simulink model "ChiefMaster_TTC580"  (R2022b)
settings: Solver=FixedStepAuto  StartTime=0.0  StopTime=10  FixedStep=0.01  RelTol=1e-3
values from neighbouring files (symbols this model uses):
  BattBox1_No = single(1)    [Parameters.m]
  BattBox2_No = single(2)    [Parameters.m]
  BattBox3_No = single(3)    [Parameters.m]
  CurrentLB = single(-3)    [Parameters.m]
  CurrentReductionConstant_Lvl0 = single(0.03)    [Parameters.m]
  CurrentReductionConstant_Lvl1 = single(0.05)    [Parameters.m]
  CurrentReductionConstant_Lvl2 = single(0.07)    [Parameters.m]
  CurrentReductionConstant_Lvl3 = single(0.1)    [Parameters.m]
  CurrentUB = single(3)    [Parameters.m]
  DCHV_Minus_In_Delay_ms = single(500)    [Parameters.m]
  FL_sHVC_CellBalanceVoltage_mV = single(3500)    [Parameters.m]
  FL_sInrushCurrent_dividebyzero = single(0.00001)    [Parameters.m]
  FL_u8HMI_BuzzerTimer = uint8(3)    [Parameters.m]
  IP_boActValue = true    [Parameters.m]
  IP_boDeactValue = false    [Parameters.m]
  IP_boInitValue = false    [Parameters.m]
  IP_s_LB = 18000    [Parameters.m]
  IP_s_UB = 22000    [Parameters.m]
  IP_sBatt1_ChargeCurrentMax_Factor = single(0.1)    [Parameters.m]
  IP_sBatt1_ChargeCurrentMax_LB = single(0)    [Parameters.m]
  IP_sBatt1_ChargeCurrentMax_Offset = single(0)    [Parameters.m]
  IP_sBatt1_ChargeCurrentMax_UB = single(6553.5)    [Parameters.m]
  IP_sBatt1_Current_Factor = single(0.1)    [Parameters.m]
  IP_sBatt1_Current_LB = single(-3276.8)    [Parameters.m]
  IP_sBatt1_Current_Offset = single(0)    [Parameters.m]
  IP_sBatt1_Current_UB = single(3276.8)    [Parameters.m]
  IP_sBatt1_DisChargeCurrentMax_Factor = single(0.1)    [Parameters.m]
  IP_sBatt1_DisChargeCurrentMax_LB = single(0)    [Parameters.m]
  IP_sBatt1_DisChargeCurrentMax_Offset = single(0)    [Parameters.m]
  IP_sBatt1_DisChargeCurrentMax_UB = single(6553.5)    [Parameters.m]
  IP_sBatt1_InsulationResistance_Factor = single(5)    [Parameters.m]
  IP_sBatt1_InsulationResistance_LB = single(0)    [Parameters.m]
  IP_sBatt1_InsulationResistance_Offset = single(0)    [Parameters.m]
  IP_sBatt1_InsulationResistance_UB = single(0)    [Parameters.m]
  IP_sBatt1_LiBa_IntResist_mOhm = single(25)    [Parameters.m]
  IP_sBatt1_SOC_Factor = single(1)    [Parameters.m]
  IP_sBatt1_SOC_LB = single(0)    [Parameters.m]
  IP_sBatt1_SOC_Offset = single(0)    [Parameters.m]
  IP_sBatt1_SOC_UB = single(100)    [Parameters.m]
  IP_sBatt1_SOH_Factor = single(1)    [Parameters.m]
  IP_sBatt1_SOH_LB = single(0)    [Parameters.m]
  IP_sBatt1_SOH_Offset = single(0)    [Parameters.m]
  IP_sBatt1_SOH_UB = single(100)    [Parameters.m]
  IP_sBatt1_Ubatt_Factor = single(0.1)    [Parameters.m]
  IP_sBatt1_Ubatt_LB = single(0)    [Parameters.m]
  IP_sBatt1_Ubatt_Offset = single(0)    [Parameters.m]
  IP_sBatt1_Ubatt_UB = single(6553.5)    [Parameters.m]
  IP_sBatt1_UserRi_Factor = single(1)    [Parameters.m]
  IP_sBatt1_UserRi_LB = single(0)    [Parameters.m]
  IP_sBatt1_UserRi_Offset = single(0)    [Parameters.m]
  IP_sBatt1_UserRi_UB = single(255)    [Parameters.m]
  IP_sBatt1_VoltageAtSensor_Factor = single(0.02)    [Parameters.m]
  IP_sBatt1_VoltageAtSensor_LB = single(0)    [Parameters.m]
  IP_sBatt1_VoltageAtSensor_Offset = single(0)    [Parameters.m]
  IP_sBatt1_VoltageAtSensor_UB = single(1310.7)    [Parameters.m]
  IP_sBatt2_LiBa_IntResist_mOhm = single(25)    [Parameters.m]
  IP_sBatt3_LiBa_IntResist_mOhm = single(25)    [Parameters.m]
  IP_sEM_LB = 2000    [Parameters.m]
  IP_sEM_UB = 8000    [Parameters.m]
  IP_sFB_LB = 5000    [Parameters.m]
  IP_sFB_UB = 10000    [Parameters.m]
  IP_sHVIL_LB = 12000    [Parameters.m]
  IP_sHVIL_UB = 15000    [Parameters.m]
  IP_sLoad_Voltage_Factor = single(1)    [Parameters.m]
  IP_sLoad_Voltage_LB = single(0)    [Parameters.m]
  IP_sLoad_Voltage_Offset = single(0)    [Parameters.m]
  IP_sLoad_Voltage_UB = single(65535)    [Parameters.m]
  IP_u8HVIL_Delay_ms = uint8(100)    [Parameters.m]
  IP_u8HW_IN_delay_ms = uint8(100)    [Parameters.m]
  IT_sInsulationSafeValue_kOhm = single(650)    [Parameters.m]
  IT_u8IMD_DelayTime_s = uint8(20)    [Parameters.m]
  MainHV_Minus_In_Delay = single(5)    [Parameters.m]
  MainHV_StatusDelay = single(5)    [Parameters.m]
  NotAvailable_uint16 = single(65535)    [Parameters.m]
  NotAvailable_uint8 = uint8(255)    [Parameters.m]
  OP_boHVIL_Supply = boolean(1)    [Parameters.m]
  SafeCurrentToCloseHV_A = single(5)    [Parameters.m]
  SafeVoltageToCloseHV_V = single(0.5)    [Parameters.m]
  UnexpectedBattChargingFcn_Available = boolean(1)    [Parameters.m]
  Voltage_NA_UB = uint16(65535)    [Parameters.m]
  VoltageSensorAvailableBB1 = boolean(0)    [Parameters.m]
  VoltageSensorAvailableBB2 = boolean(0)    [Parameters.m]
  VoltageSensorAvailableBB3 = boolean(0)    [Parameters.m]
libraries: simulink x184, Library_DataProcessing_v1_1 x167, Library_DataProcessing_v1 x142, libCM x28
(part 6 of 19)

== system ChiefMaster_TTC580/ChiefMaster/Flow Logic/System Status/Subsystem1 ==
  IP_boBMS_SDError_BB1 : Inport
  IP_boBMS_SDError_BB2 : Inport  Port=2
  IP_boBMS_SDError_BB3 : Inport  Port=3
  IP_boBMS_HV_REL_ON_BB1 : Inport  Port=4
  IP_boBMS_HV_REL_ON_BB2 : Inport  Port=5
  IP_boBMS_HV_REL_ON_BB3 : Inport  Port=6
  Add : Sum  Inputs=++++++
  Constant : Constant  Value=0  OutDataTypeStr=boolean
  Constant1 : Constant  Value=0  OutDataTypeStr=boolean
  OR : Logic  Operator=OR  Inputs=3  AllPortsSameDT=off  OutDataTypeStr=boolean
  Switch : Switch  Criteria=u2 > Threshold  SaturateOnIntegerOverflow=off  InputSameDT=off
  Switch1 : Switch  Criteria=u2 > Threshold  SaturateOnIntegerOverflow=off  InputSameDT=off
  Switch2 : Switch  Criteria=u2 > Threshold  SaturateOnIntegerOverflow=off  InputSameDT=off
  FL_boSS_System_Error : Outport
  FL_u8SS_System_ErrorCode : Outport  Port=2
  wires:
  IP_boBMS_SDError_BB1/1 -> Switch/1
  IP_boBMS_SDError_BB2/1 -> Switch1/1
  IP_boBMS_SDError_BB3/1 -> Switch2/1
  OR/1 -> FL_boSS_System_Error/1  "FL_boSS_System_Error"
  IP_boBMS_HV_REL_ON_BB1/1 -> Switch/2
  Constant/1 -> Switch/3, Switch2/3, Switch1/3
  IP_boBMS_HV_REL_ON_BB2/1 -> Switch1/2
  IP_boBMS_HV_REL_ON_BB3/1 -> Switch2/2
  Add/1 -> FL_u8SS_System_ErrorCode/1  "FL_u8SS_System_ErrorCode"
  Switch2/1 -> Add/3, OR/3
  Switch/1 -> Add/1, OR/1
  Constant1/1 -> Add/4, Add/5, Add/6
  Switch1/1 -> Add/2, OR/2

== system ChiefMaster_TTC580/ChiefMaster/Flow Logic/System Status/Subsystem2 ==
  BatteryPackSignals : Inport
  Bus Selector : BusSelector  OutputSignals=IT_BatterySignal_Databus.IT_u8BMS_SOC_BB1,IT_BatterySignal_Databus.IT_boBMS_HV_REL_ON_BB1,IT_BatterySignal_Databus.IT_u8BMS_SOC_BB2,IT_BatterySignal_Databus.IT_boBMS_HV_REL_ON_BB2,IT_BatterySignal_Databus.IT_u8BMS_SOC_BB3,IT_BatterySignal_Databus.IT_boBMS_HV_REL_ON_BB3
  Constant : Constant  Value=NotAvailable_uint8  OutDataTypeStr=uint8
  Constant1 : Constant  Value=0  OutDataTypeStr=uint8
  Data Type Conversion : DataTypeConversion  OutDataTypeStr=uint8  SaturateOnIntegerOverflow=off  RndMeth=Floor
  Data Type Conversion1 : DataTypeConversion  OutDataTypeStr=uint8  SaturateOnIntegerOverflow=off  RndMeth=Floor
  Data Type Conversion2 : DataTypeConversion  OutDataTypeStr=uint8  SaturateOnIntegerOverflow=off  RndMeth=Floor
  Min : MinMax  Inputs=3
  OR : Logic  Operator=OR  Inputs=3  AllPortsSameDT=off  OutDataTypeStr=boolean
  Switch{,1..3} (4 alike) : Switch  Criteria=u2 > Threshold  SaturateOnIntegerOverflow=off  InputSameDT=off
  FL_u8SS_SystemSOC : Outport
  wires:
  Min/1 -> FL_u8SS_SystemSOC/1
  Bus Selector/6 -> OR/1, Switch2/2  "<IT_boBMS_HV_REL_ON_BB3>"
  Bus Selector/2 -> OR/3, Switch/2  "<IT_boBMS_HV_REL_ON_BB1>"
  Bus Selector/4 -> OR/2, Switch1/2  "<IT_boBMS_HV_REL_ON_BB2>"
  Switch2/1 -> Min/3
  Switch/1 -> Min/1
  Bus Selector/1 -> Data Type Conversion/1  "<IT_u8BMS_SOC_BB1>"
  Switch1/1 -> Min/2
  Bus Selector/3 -> Data Type Conversion1/1  "<IT_u8BMS_SOC_BB2>"
  Bus Selector/5 -> Data Type Conversion2/1  "<IT_u8BMS_SOC_BB3>"
  Switch3/1 -> Switch2/3, Switch/3, Switch1/3
  OR/1 -> Switch3/2
  Constant/1 -> Switch3/1
  Constant1/1 -> Switch3/3
  BatteryPackSignals/1 -> Bus Selector/1
  Data Type Conversion/1 -> Switch/1
  Data Type Conversion1/1 -> Switch1/1
  Data Type Conversion2/1 -> Switch2/1

== system ChiefMaster_TTC580/ChiefMaster/Flow Logic/System Status/Subsystem3 ==
  BatteryPackSignals : Inport
  Add : Sum  Inputs=+++
  Bus Selector : BusSelector  OutputSignals=IT_BatterySignal_Databus.IT_sBMS_Current_BB1,IT_BatterySignal_Databus.IT_sBMS_Current_BB2,IT_BatterySignal_Databus.IT_sBMS_Current_BB3
  FL_sSS_System_Current : Outport
  wires:
  Bus Selector/3 -> Add/3  "<IT_sBMS_Current_BB3>"
  Bus Selector/2 -> Add/2  "<IT_sBMS_Current_BB2>"
  Bus Selector/1 -> Add/1  "<IT_sBMS_Current_BB1>"
  Add/1 -> FL_sSS_System_Current/1
  BatteryPackSignals/1 -> Bus Selector/1

== system ChiefMaster_TTC580/ChiefMaster/Flow Logic/System Status/Subsystem4 ==
  BatteryPackSignals : Inport
  Bus Selector : BusSelector  OutputSignals=IT_BatterySignal_Databus.IT_sBMS_VtgInt_BB1,IT_BatterySignal_Databus.IT_boBMS_HV_REL_ON_BB1,IT_BatterySignal_Databus.IT_sBMS_VtgInt_BB2,IT_BatterySignal_Databus.IT_boBMS_HV_REL_ON_BB2,IT_BatterySignal_Databus.IT_sBMS_VtgInt_BB3,IT_BatterySignal_Databus.IT_boBMS_HV_REL_ON_BB3
  Constant : Constant  Value=0  OutDataTypeStr=single
  Min : MinMax  Function=max  Inputs=3
  Switch : Switch  Criteria=u2 > Threshold  SaturateOnIntegerOverflow=off  InputSameDT=off
  Switch1 : Switch  Criteria=u2 > Threshold  SaturateOnIntegerOverflow=off  InputSameDT=off
  Switch2 : Switch  Criteria=u2 > Threshold  SaturateOnIntegerOverflow=off  InputSameDT=off
  FL_sST_SystemVoltage : Outport
  wires:
  BatteryPackSignals/1 -> Bus Selector/1
  Min/1 -> FL_sST_SystemVoltage/1
  Bus Selector/6 -> Switch2/2  "<IT_boBMS_HV_REL_ON_BB3>"
  Bus Selector/2 -> Switch/2  "<IT_boBMS_HV_REL_ON_BB1>"
  Bus Selector/4 -> Switch1/2  "<IT_boBMS_HV_REL_ON_BB2>"
  Switch2/1 -> Min/3
  Switch/1 -> Min/1
  Bus Selector/1 -> Switch/1  "<IT_sBMS_VtgInt_BB1>"
  Switch1/1 -> Min/2
  Bus Selector/3 -> Switch1/1  "<IT_sBMS_VtgInt_BB2>"
  Bus Selector/5 -> Switch2/1  "<IT_sBMS_VtgInt_BB3>"
  Constant/1 -> Switch/3, Switch1/3, Switch2/3

== system ChiefMaster_TTC580/ChiefMaster/Flow Logic/System Status/Subsystem7 ==
  IP_boBMS_HV_REL_ON_BB1 : Inport
  IP_boBMS_HV_REL_ON_BB2 : Inport  Port=2
  IP_boBMS_HV_REL_ON_BB3 : Inport  Port=3
  FL_u8Sig_No_Of_Batt_Usable : Inport  Port=4
  IP_boBMS_SDError_BB1 : Inport  Port=5
  IP_boBMS_SDError_BB2 : Inport  Port=6
  IP_boBMS_SDError_BB3 : Inport  Port=7
  AND : Logic  Inputs=4  AllPortsSameDT=off  OutDataTypeStr=boolean
  AND1 : Logic  Inputs=4  AllPortsSameDT=off  OutDataTypeStr=boolean
  AND2 : Logic  Inputs=4  AllPortsSameDT=off  OutDataTypeStr=boolean
  Add : Sum  Inputs=+++
  Compare To Constant : simulink/Logic and Bit Operations/Compare To Constant  relop===  const=1  OutDataTypeStr=boolean
  Compare To Constant1 : simulink/Logic and Bit Operations/Compare To Constant  relop=>  const=0  OutDataTypeStr=boolean
  OR3 : Logic  Operator=OR  Inputs=3  AllPortsSameDT=off  OutDataTypeStr=boolean
  Unit Delay : UnitDelay  SampleTime=-1  HasFrameUpgradeWarning=on
  Unit Delay1 : UnitDelay  SampleTime=-1  HasFrameUpgradeWarning=on
  Unit Delay2 : UnitDelay  SampleTime=-1  HasFrameUpgradeWarning=on
  FL_u8SS_NumberOfConnectedBatt : Outport
  FL_boSS_BDU_Reset : Outport  Port=2
  wires:
  Compare To Constant1/1 -> AND2/3, AND1/1, AND/3
  AND/1 -> OR3/1  "BDU_Reset"
  Compare To Constant/1 -> AND1/2, AND2/2, AND/2
  AND2/1 -> OR3/3  "BDU_Reset"
  Unit Delay1/1 -> AND1/4
  IP_boBMS_HV_REL_ON_BB2/1 -> Add/2, AND1/3
  FL_u8Sig_No_Of_Batt_Usable/1 -> Compare To Constant1/1
  IP_boBMS_HV_REL_ON_BB1/1 -> Add/1, AND/1
  Add/1 -> FL_u8SS_NumberOfConnectedBatt/1, Compare To Constant/1  "FL_u8SS_NumberOfConnectedBatt"
  IP_boBMS_HV_REL_ON_BB3/1 -> AND2/1, Add/3
  AND1/1 -> OR3/2  "BDU_Reset"
  Unit Delay/1 -> AND/4
  Unit Delay2/1 -> AND2/4
  OR3/1 -> FL_boSS_BDU_Reset/1  "FL_boSS_BDU_Reset"
  IP_boBMS_SDError_BB3/1 -> Unit Delay2/1
  IP_boBMS_SDError_BB1/1 -> Unit Delay/1
  IP_boBMS_SDError_BB2/1 -> Unit Delay1/1

== system ChiefMaster_TTC580/ChiefMaster/Flow Logic/System Status/Subsystem8 ==
  <FL_boREQ_IMD_ON_BB1> : Inport
  <FL_boREQ_IMD_ON_BB2> : Inport  Port=2
  <FL_boREQ_IMD_ON_BB3> : Inport  Port=3
  AND : Logic  Inputs=3  AllPortsSameDT=off  OutDataTypeStr=boolean
  Unit Delay7 : UnitDelay  SampleTime=-1  HasFrameUpgradeWarning=on
  Unit Delay8 : UnitDelay  SampleTime=-1  HasFrameUpgradeWarning=on
  Unit Delay9 : UnitDelay  SampleTime=-1  HasFrameUpgradeWarning=on
  REQ_IMD_ON : Outport
  wires:
  <FL_boREQ_IMD_ON_BB3>/1 -> Unit Delay7/1
  <FL_boREQ_IMD_ON_BB1>/1 -> Unit Delay9/1
  <FL_boREQ_IMD_ON_BB2>/1 -> Unit Delay8/1
  AND/1 -> REQ_IMD_ON/1
  Unit Delay9/1 -> AND/1
  Unit Delay8/1 -> AND/2
  Unit Delay7/1 -> AND/3

== system ChiefMaster_TTC580/ChiefMaster/Input Processing/Actia/Batt Box 1 ==
  C_Actia_Batt1_MyStatus : Inport
  C_Actia_Batt1_MyStatus_Timeout : Inport  Port=2  OutDataTypeStr=boolean
  C_Actia_Batt1_Error : Inport  Port=3
  C_Actia_Batt1_Error_Timeout : Inport  Port=4  OutDataTypeStr=boolean
  C_Actia_Batt1_ADS_8 : Inport  Port=5
  C_Actia_Batt1_ADS_8_Timeout : Inport  Port=6  OutDataTypeStr=boolean
  C_Actia_Batt1_ADS_0 : Inport  Port=7
  C_Actia_Batt1_ADS_0_Timeout : Inport  Port=8
  C_Actia_Batt1_ADS_1 : Inport  Port=9
  C_Actia_Batt1_ADS_1_Timeout : Inport  Port=10  OutDataTypeStr=boolean
  C_Actia_Batt1_ADS_3 : Inport  Port=11
  C_Actia_Batt1_ADS_3_Timeout : Inport  Port=12
  Bus Creator : BusCreator  Inputs=17
  Subsystem1 : Subsystem
  Subsystem13 : Subsystem
  Subsystem2 : Subsystem
  Subsystem3 : Subsystem
  Subsystem4 : Subsystem
  Subsystem5 : Subsystem
  Subsystem6 : Subsystem
  IP_Actia_Batt1_Databus : Outport
  wires:
  Subsystem2/3(IP_sActia_Batt1_DisChargeCurrentMax_A_Databus) -> Bus Creator/3
  Subsystem5/3(IP_sActia_Batt1_SOC_percent_DataBus) -> Bus Creator/9
  Subsystem4/1(IP_Actia_sBatt1_MyStatus2_Databus) -> Bus Creator/5
  C_Actia_Batt1_ADS_1_Timeout/1 -> Subsystem13/5(C_Batt1_ADS_1_520_Timeout), Subsystem6/2(C_Batt1_ADS_1_520_Timeout)
  C_Actia_Batt1_MyStatus_Timeout/1 -> Subsystem13/1(C_Batt1_MyStatus_140_Timeout), Subsystem2/2(C_Actia_Batt1_MyStatus_Timeout)
  C_Actia_Batt1_ADS_1/1 -> Subsystem6/1(C_Batt1_ADS_1_520)
  C_Actia_Batt1_ADS_3_Timeout/1 -> Subsystem13/6(C_Batt1_ADS_3_560_Timeout), Subsystem1/2(C_Batt1_ADS_3_560_Timeout)
  C_Actia_Batt1_Error_Timeout/1 -> Subsystem4/2(C_Actia_Batt1_Error_Timeout), Subsystem13/2(C_Batt1_Error_100_Timeout)
  C_Actia_Batt1_ADS_8/1 -> Subsystem5/1(C_Batt1_ADS_8_600)
  Subsystem6/1(IP_sActia_Batt1_UserRi_mOhms_DataBus) -> Bus Creator/13
  Subsystem1/1(IP_sActia_Batt1_Ubatt_Databus) -> Bus Creator/16
  Subsystem5/2(IP_sActia_Batt1_InsulationResistance_kOhms_DataBus) -> Bus Creator/8
  Subsystem2/4(IP_sActia_Batt1_VoltageAtSensor_V_Databus) -> Bus Creator/4
  Subsystem2/2(IP_sActia_Batt1_ChargeCurrentMax_A_Databus) -> Bus Creator/2
  C_Actia_Batt1_ADS_8_Timeout/1 -> Subsystem13/3(C_Batt1_ADS_8_600_Timeout), Subsystem5/2(C_Batt1_ADS_8_600_Timeout)
  Subsystem5/1(IP_sActia_Batt1_Current_A_DataBus) -> Bus Creator/7
  Subsystem5/4(IP_sActia_Batt1_SOH_percent_DataBus) -> Bus Creator/10
  Subsystem2/1(Batt1_MyStatus1_Databus) -> Bus Creator/1
  Subsystem13/1(IP_sActia_Batt1_Availability) -> Bus Creator/17
  Bus Creator/1 -> IP_Actia_Batt1_Databus/1  "IP_Actia_Batt1_Databus"
  C_Actia_Batt1_ADS_3/1 -> Subsystem1/1(C_Batt1_ADS_3_560)
  C_Actia_Batt1_MyStatus/1 -> Subsystem2/1(C_Actia_Batt1_MyStatus_Msg)
  C_Actia_Batt1_Error/1 -> Subsystem4/1(C_Actia_Batt1_Error)
  Subsystem4/2(IP_Actia_Batt1_Error_Databus) -> Bus Creator/6
  Subsystem6/2(IP_sActia_Batt1_MinTemp_degC_DataBus) -> Bus Creator/14
  Subsystem6/3(IP_sActia_Batt1_MaxTemp_degC_DataBus) -> Bus Creator/15
  C_Actia_Batt1_ADS_0/1 -> Subsystem3/1(C_Batt1_ADS_0_500)
  C_Actia_Batt1_ADS_0_Timeout/1 -> Subsystem13/4(C_Batt1_ADS_0_500_Timeout), Subsystem3/2(C_Batt1_ADS_0_500_Timeout)
  Subsystem3/1(IP_sActia_Batt1_MinCellVolt_mV_DataBus) -> Bus Creator/11
  Subsystem3/2(IP_sActia_Batt1_MaxCellVolt_mV_DataBus) -> Bus Creator/12

== system ChiefMaster_TTC580/ChiefMaster/Input Processing/Actia/Batt Box 2 ==
  C_Actia_Batt2_MyStatus : Inport
  C_Actia_Batt2_MyStatus_Timeout : Inport  Port=2  OutDataTypeStr=boolean
  C_Actia_Batt2_Error : Inport  Port=3
  C_Actia_Batt2_Error_Timeout : Inport  Port=4  OutDataTypeStr=boolean
  C_Actia_Batt2_ADS_8 : Inport  Port=5
  C_Actia_Batt2_ADS_8_Timeout : Inport  Port=6  OutDataTypeStr=boolean
  C_Actia_Batt2_ADS_0 : Inport  Port=7
  C_Actia_Batt2_ADS_0_Timeout : Inport  Port=8
  C_Actia_Batt2_ADS_1 : Inport  Port=9
  C_Actia_Batt2_ADS_1_Timeout : Inport  Port=10  OutDataTypeStr=boolean
  C_Actia_Batt2_ADS_3 : Inport  Port=11
  C_Actia_Batt2_ADS_3_Timeout : Inport  Port=12
  Bus Creator : BusCreator  Inputs=17
  Subsystem1 : Subsystem
  Subsystem13 : Subsystem
  Subsystem2 : Subsystem
  Subsystem3 : Subsystem
  Subsystem4 : Subsystem
  Subsystem5 : Subsystem
  Subsystem6 : Subsystem
  IP_Actia_Batt2_Databus : Outport
  wires:
  Subsystem4/2(IP_Actia_Batt2_Error_Databus) -> Bus Creator/6
  C_Actia_Batt2_Error/1 -> Subsystem4/1(C_Actia_Batt2_Error)
  C_Actia_Batt2_MyStatus/1 -> Subsystem2/1(C_Actia_Batt2_MyStatus_Msg)
  C_Actia_Batt2_ADS_3/1 -> Subsystem1/1(C_Batt2_ADS_3_560)
  Bus Creator/1 -> IP_Actia_Batt2_Databus/1  "IP_Actia_Batt2_Databus"
  Subsystem13/1(IP_sActia_Batt2_Availability) -> Bus Creator/17
  Subsystem2/1(Batt2_MyStatus1_Databus) -> Bus Creator/1
  Subsystem5/4(IP_sActia_Batt2_SOH_percent_DataBus) -> Bus Creator/10
  Subsystem5/1(IP_sActia_Batt2_Current_A_DataBus) -> Bus Creator/7
  C_Actia_Batt2_ADS_8_Timeout/1 -> Subsystem5/2(C_Batt2_ADS_8_600_Timeout), Subsystem13/3(C_Batt2_ADS_8_600_Timeout)
  Subsystem2/2(IP_sActia_Batt2_ChargeCurrentMax_A_Databus) -> Bus Creator/2
  Subsystem2/4(IP_sActia_Batt2_VoltageAtSensor_V_Databus) -> Bus Creator/4
  Subsystem5/2(IP_sActia_Batt2_InsulationResistance_kOhms_DataBus) -> Bus Creator/8
  Subsystem1/1(IP_sActia_Batt2_Ubatt_Databus) -> Bus Creator/16
  Subsystem6/1(IP_sActia_Batt2_UserRi_mOhms_DataBus) -> Bus Creator/13
  C_Actia_Batt2_ADS_8/1 -> Subsystem5/1(C_Batt2_ADS_8_600)
  C_Actia_Batt2_Error_Timeout/1 -> Subsystem4/2(C_Actia_Batt2_Error_Timeout), Subsystem13/2(C_Batt2_Error_100_Timeout)
  C_Actia_Batt2_ADS_3_Timeout/1 -> Subsystem1/2(C_Batt2_ADS_3_560_Timeout), Subsystem13/6(C_Batt2_ADS_3_560_Timeout)
  C_Actia_Batt2_ADS_1/1 -> Subsystem6/1(C_Batt2_ADS_1_520)
  C_Actia_Batt2_MyStatus_Timeout/1 -> Subsystem2/2(C_Actia_Batt2_MyStatus_Timeout), Subsystem13/1(C_Batt2_MyStatus_140_Timeout)
  C_Actia_Batt2_ADS_1_Timeout/1 -> Subsystem6/2(C_Batt2_ADS_1_520_Timeout), Subsystem13/5(C_Batt2_ADS_1_520_Timeout)
  Subsystem4/1(IP_Actia_sBatt2_MyStatus2_Databus) -> Bus Creator/5
  Subsystem5/3(IP_sActia_Batt2_SOC_percent_DataBus) -> Bus Creator/9
  Subsystem2/3(IP_sActia_Batt2_DisChargeCurrentMax_A_Databus) -> Bus Creator/3
  Subsystem6/2(IP_sActia_Batt2_MinTemp_degC_DataBus) -> Bus Creator/14
  Subsystem6/3(IP_sActia_Batt2_MaxTemp_degC_DataBus) -> Bus Creator/15
  C_Actia_Batt2_ADS_0_Timeout/1 -> Subsystem13/4(C_Batt2_ADS_501_Timeout), Subsystem3/2(C_Batt1_ADS_0_500_Timeout)
  Subsystem3/2(IP_sActia_Batt2_MaxCellVolt_mV_DataBus) -> Bus Creator/12
  Subsystem3/1(IP_sActia_Batt2_MinCellVolt_mV_DataBus) -> Bus Creator/11
  C_Actia_Batt2_ADS_0/1 -> Subsystem3/1(C_Batt1_ADS_0_500)

== system ChiefMaster_TTC580/ChiefMaster/Input Processing/Actia/Batt Box 3 ==
  C_Actia_Batt3_MyStatus : Inport
  C_Actia_Batt3_MyStatus_Timeout : Inport  Port=2
  C_Actia_Batt3_Error : Inport  Port=3
  C_Actia_Batt3_Error_Timeout : Inport  Port=4
  C_Actia_Batt3_ADS_8 : Inport  Port=5
  C_Actia_Batt3_ADS_8_Timeout : Inport  Port=6
  C_Actia_Batt3_ADS_0 : Inport  Port=7
  C_Actia_Batt3_ADS_0_Timeout : Inport  Port=8
  C_Actia_Batt3_ADS_1 : Inport  Port=9
  C_Actia_Batt3_ADS_1_Timeout : Inport  Port=10
  C_Actia_Batt3_ADS_3 : Inport  Port=11
  C_Actia_Batt3_ADS_3_Timeout : Inport  Port=12
  Bus Creator : BusCreator  Inputs=17
  Subsystem1 : Subsystem
  Subsystem13 : Subsystem
  Subsystem2 : Subsystem
  Subsystem3 : Subsystem
  Subsystem4 : Subsystem
  Subsystem5 : Subsystem
  Subsystem6 : Subsystem
  IP_Actia_Batt3_Databus : Outport
  wires:
  Subsystem2/3(IP_sActia_Batt3_DisChargeCurrentMax_A_Databus) -> Bus Creator/3
  Subsystem5/3(IP_sActia_Batt3_SOC_percent_DataBus) -> Bus Creator/9
  Subsystem4/1(IP_Actia_sBatt3_MyStatus2_Databus) -> Bus Creator/5
  C_Actia_Batt3_ADS_1_Timeout/1 -> Subsystem13/5(C_Batt3_ADS_1_520_Timeout), Subsystem6/2(C_Batt3_ADS_1_520_Timeout)
  C_Actia_Batt3_MyStatus_Timeout/1 -> Subsystem13/1(C_Batt3_MyStatus_140_Timeout), Subsystem2/2(C_Actia_Batt3_MyStatus_Timeout)
  C_Actia_Batt3_ADS_1/1 -> Subsystem6/1(C_Batt3_ADS_1_520)
  C_Actia_Batt3_ADS_3_Timeout/1 -> Subsystem13/6(C_Batt3_ADS_3_560_Timeout), Subsystem1/2(C_Batt3_ADS_3_560_Timeout)
  C_Actia_Batt3_Error_Timeout/1 -> Subsystem4/2(C_Actia_Batt3_Error_Timeout), Subsystem13/2(C_Batt3_Error_100_Timeout)
  C_Actia_Batt3_ADS_8/1 -> Subsystem5/1(C_Batt3_ADS_8_600)
  Subsystem6/1(IP_sActia_Batt3_UserRi_mOhms_DataBus) -> Bus Creator/13
  Subsystem1/1(IP_sActia_Batt3_Ubatt_Databus) -> Bus Creator/16
  Subsystem5/2(IP_sActia_Batt3_InsulationResistance_kOhms_DataBus) -> Bus Creator/8
  Subsystem2/4(IP_sActia_Batt3_VoltageAtSensor_V_Databus) -> Bus Creator/4
  Subsystem2/2(IP_sActia_Batt3_ChargeCurrentMax_A_Databus) -> Bus Creator/2
  C_Actia_Batt3_ADS_8_Timeout/1 -> Subsystem5/2(C_Batt3_ADS_8_600_Timeout), Subsystem13/3(C_Batt3_ADS_8_600_Timeout)
  Subsystem5/1(IP_sActia_Batt3_Current_A_DataBus) -> Bus Creator/7
  Subsystem5/4(IP_sActia_Batt3_SOH_percent_DataBus) -> Bus Creator/10
  Subsystem2/1(Batt3_MyStatus1_Databus) -> Bus Creator/1
  Subsystem13/1(IP_sActia_Batt3_Availability) -> Bus Creator/17
  Bus Creator/1 -> IP_Actia_Batt3_Databus/1  "IP_Actia_Batt3_Databus"
  C_Actia_Batt3_ADS_3/1 -> Subsystem1/1(C_Batt3_ADS_3_560)
  C_Actia_Batt3_MyStatus/1 -> Subsystem2/1(C_Actia_Batt3_MyStatus_Msg)
  C_Actia_Batt3_Error/1 -> Subsystem4/1(C_Actia_Batt3_Error)
  Subsystem4/2(IP_Actia_Batt3_Error_Databus) -> Bus Creator/6
  Subsystem6/2(IP_sActia_Batt3_MinTemp_degC_DataBus) -> Bus Creator/14
  Subsystem6/3(IP_sActia_Batt3_MaxTemp_degC_DataBus) -> Bus Creator/15
  C_Actia_Batt3_ADS_0_Timeout/1 -> Subsystem13/4(C_Batt2_ADS_0_Timeout), Subsystem3/2(C_Batt1_ADS_0_500_Timeout)
  C_Actia_Batt3_ADS_0/1 -> Subsystem3/1(C_Batt1_ADS_0_500)
  Subsystem3/1(IP_sActia_Batt3_MinCellVolt_mV_DataBus) -> Bus Creator/11
  Subsystem3/2(IP_sActia_Batt3_MaxCellVolt_mV_DataBus) -> Bus Creator/12

== system ChiefMaster_TTC580/ChiefMaster/Input Processing/HW Inputs/EmergencyButtonNC ==
  "EmergencyButton_NC " : Inport  OutDataTypeStr=single
  Constant : Constant  Value=IP_sEM_LB  OutDataTypeStr=single
  Constant1 : Constant  Value=IP_sEM_UB  OutDataTypeStr=single
  Constant2 : Constant  Value=IP_boActValue  OutDataTypeStr=boolean
  Constant3 : Constant  Value=IP_boDeactValue  OutDataTypeStr=boolean
  Constant4 : Constant  Value=IP_boInitValue  OutDataTypeStr=boolean
  Lib_Hysteresis_HighActive : Library_DataProcessing_v1_1/Lib_Hysteresis_HighActive  SystemSampleTime=-1  VariantActivationTime=update diagram  Latency=0  AutoFrameSizeCalculation=off
  IP_boHW_EmergencyButton_NC : Outport
  wires:
  Lib_Hysteresis_HighActive/1 -> IP_boHW_EmergencyButton_NC/1  "IP_boHW_EmergencyButton_NC"
  Constant1/1 -> Lib_Hysteresis_HighActive/6
  Constant/1 -> Lib_Hysteresis_HighActive/5
  Constant3/1 -> Lib_Hysteresis_HighActive/4
  Constant2/1 -> Lib_Hysteresis_HighActive/3
  Constant4/1 -> Lib_Hysteresis_HighActive/2
  "EmergencyButton_NC "/1 -> Lib_Hysteresis_HighActive/1

== system ChiefMaster_TTC580/ChiefMaster/Input Processing/HW Inputs/EmergencyButtonNO ==
  "EmergencyButton_NO " : Inport  OutDataTypeStr=single
  Constant : Constant  Value=IP_s_UB  OutDataTypeStr=single
  Constant1 : Constant  Value=IP_s_LB  OutDataTypeStr=single
  Constant2 : Constant  Value=IP_boActValue  OutDataTypeStr=boolean
  Constant3 : Constant  Value=IP_boDeactValue  OutDataTypeStr=boolean
  Constant4 : Constant  Value=IP_boInitValue  OutDataTypeStr=boolean
  Lib_Hysteresis_HighActive : Library_DataProcessing_v1_1/Lib_Hysteresis_HighActive  SystemSampleTime=-1  VariantActivationTime=update diagram  Latency=0  AutoFrameSizeCalculation=off
  IP_boHW_EmergencyButton_NO : Outport
  wires:
  "EmergencyButton_NO "/1 -> Lib_Hysteresis_HighActive/1
  Constant4/1 -> Lib_Hysteresis_HighActive/2
  Constant2/1 -> Lib_Hysteresis_HighActive/3
  Constant3/1 -> Lib_Hysteresis_HighActive/4
  Constant/1 -> Lib_Hysteresis_HighActive/6
  Constant1/1 -> Lib_Hysteresis_HighActive/5
  Lib_Hysteresis_HighActive/1 -> IP_boHW_EmergencyButton_NO/1  "IP_boHW_EmergencyButton_NO"

== system ChiefMaster_TTC580/ChiefMaster/Input Processing/HW Inputs/HVIL ==
  IP_sHW_HVIL_BDU : Inport
  Constant : Constant  Value=IP_sHVIL_UB  OutDataTypeStr=single
  Constant1 : Constant  Value=IP_sHVIL_LB  OutDataTypeStr=single
  Constant2 : Constant  Value=IP_boActValue  OutDataTypeStr=boolean
  Constant3 : Constant  Value=IP_boDeactValue  OutDataTypeStr=boolean
  Constant4 : Constant  Value=IP_boInitValue  OutDataTypeStr=boolean
  Constant5 : Constant  Value=IP_u8HVIL_Delay_ms  OutDataTypeStr=uint8
  HVIL_Input_Delay : Stateflow chart  TreatAsAtomicUnit=on
  Lib_Hysteresis_HighActive : Library_DataProcessing_v1_1/Lib_Hysteresis_HighActive  SystemSampleTime=-1  VariantActivationTime=update diagram  Latency=0  AutoFrameSizeCalculation=off
  IP_boHW_HVIL_BDU : Outport
  wires:
  Constant4/1 -> Lib_Hysteresis_HighActive/2
  Constant2/1 -> Lib_Hysteresis_HighActive/3
  Constant3/1 -> Lib_Hysteresis_HighActive/4
  Constant1/1 -> Lib_Hysteresis_HighActive/5
  Constant/1 -> Lib_Hysteresis_HighActive/6
  IP_sHW_HVIL_BDU/1 -> Lib_Hysteresis_HighActive/1
  HVIL_Input_Delay/1(out) -> IP_boHW_HVIL_BDU/1  "IP_boHW_HVIL_BDU"
  Lib_Hysteresis_HighActive/1 -> HVIL_Input_Delay/1(HVIL_IN)  "IP_boHW_HVIL_BDU"
  Constant5/1 -> HVIL_Input_Delay/2(IP_HVIL_Delay_ms)

== system ChiefMaster_TTC580/ChiefMaster/Input Processing/HW Inputs/HVIL1 ==
  IP_sHW_HVIL_BDU : Inport
  Constant : Constant  Value=IP_sHVIL_UB  OutDataTypeStr=single
  Constant1 : Constant  Value=IP_sHVIL_LB  OutDataTypeStr=single
  Constant2 : Constant  Value=IP_boActValue  OutDataTypeStr=boolean
  Constant3 : Constant  Value=IP_boDeactValue  OutDataTypeStr=boolean
  Constant4 : Constant  Value=IP_boInitValue  OutDataTypeStr=boolean
  Constant5 : Constant  Value=IP_u8HVIL_Delay_ms  OutDataTypeStr=uint8
  HVIL_Input_Delay : Stateflow chart  TreatAsAtomicUnit=on
  Lib_Hysteresis_HighActive : Library_DataProcessing_v1_1/Lib_Hysteresis_HighActive  SystemSampleTime=-1  VariantActivationTime=update diagram  Latency=0  AutoFrameSizeCalculation=off
  IP_boHW_HVIL_Components : Outport
  wires:
  HVIL_Input_Delay/1(out) -> IP_boHW_HVIL_Components/1  "IP_boHW_HVIL_Components"
  IP_sHW_HVIL_BDU/1 -> Lib_Hysteresis_HighActive/1
  Constant4/1 -> Lib_Hysteresis_HighActive/2
  Constant1/1 -> Lib_Hysteresis_HighActive/5
  Constant3/1 -> Lib_Hysteresis_HighActive/4
  Constant2/1 -> Lib_Hysteresis_HighActive/3
  Constant/1 -> Lib_Hysteresis_HighActive/6
  Lib_Hysteresis_HighActive/1 -> HVIL_Input_Delay/1(HVIL_IN)  "IP_boHW_HVIL_Components"
  Constant5/1 -> HVIL_Input_Delay/2(IP_HVIL_Delay_ms)

== system ChiefMaster_TTC580/ChiefMaster/Input Processing/HW Inputs/HVIL2 ==
  IP_sHW_HVIL_BDU : Inport
  Constant : Constant  Value=IP_sHVIL_UB  OutDataTypeStr=single
  Constant1 : Constant  Value=IP_sHVIL_LB  OutDataTypeStr=single
  Constant2 : Constant  Value=IP_boActValue  OutDataTypeStr=boolean
  Constant3 : Constant  Value=IP_boDeactValue  OutDataTypeStr=boolean
  Constant4 : Constant  Value=IP_boInitValue  OutDataTypeStr=boolean
  Constant5 : Constant  Value=IP_u8HVIL_Delay_ms  OutDataTypeStr=uint8
  HVIL_Input_Delay : Stateflow chart  TreatAsAtomicUnit=on
  Lib_Hysteresis_HighActive : Library_DataProcessing_v1_1/Lib_Hysteresis_HighActive  SystemSampleTime=-1  VariantActivationTime=update diagram  Latency=0  AutoFrameSizeCalculation=off
  IP_boHW_HVIL_Battery : Outport
  wires:
  IP_sHW_HVIL_BDU/1 -> Lib_Hysteresis_HighActive/1
  HVIL_Input_Delay/1(out) -> IP_boHW_HVIL_Battery/1  "IP_boHW_HVIL_Battery"
  Constant4/1 -> Lib_Hysteresis_HighActive/2
  Constant1/1 -> Lib_Hysteresis_HighActive/5
  Constant3/1 -> Lib_Hysteresis_HighActive/4
  Constant2/1 -> Lib_Hysteresis_HighActive/3
  Constant/1 -> Lib_Hysteresis_HighActive/6
  Lib_Hysteresis_HighActive/1 -> HVIL_Input_Delay/1(HVIL_IN)  "IP_boHW_HVIL_Battery"
  Constant5/1 -> HVIL_Input_Delay/2(IP_HVIL_Delay_ms)

== system ChiefMaster_TTC580/ChiefMaster/Input Processing/HW Inputs/Ignition ==
  "AI_KL15 " : Inport  OutDataTypeStr=single
  Constant : Constant  Value=IP_s_UB  OutDataTypeStr=single
  Constant1 : Constant  Value=IP_s_LB  OutDataTypeStr=single
  Constant2 : Constant  Value=IP_boActValue  OutDataTypeStr=boolean
  Constant3 : Constant  Value=IP_boDeactValue  OutDataTypeStr=boolean
  Constant4 : Constant  Value=IP_boInitValue  OutDataTypeStr=boolean
  Lib_Hysteresis_HighActive : Library_DataProcessing_v1_1/Lib_Hysteresis_HighActive  SystemSampleTime=-1  VariantActivationTime=update diagram  Latency=0  AutoFrameSizeCalculation=off
  IP_boHW_KL15 : Outport
  wires:
  Lib_Hysteresis_HighActive/1 -> IP_boHW_KL15/1  "IP_boHW_KL15"
  "AI_KL15 "/1 -> Lib_Hysteresis_HighActive/1
  Constant/1 -> Lib_Hysteresis_HighActive/6
  Constant1/1 -> Lib_Hysteresis_HighActive/5
  Constant3/1 -> Lib_Hysteresis_HighActive/4
  Constant2/1 -> Lib_Hysteresis_HighActive/3
  Constant4/1 -> Lib_Hysteresis_HighActive/2

== system ChiefMaster_TTC580/ChiefMaster/Input Processing/HW Inputs/Minus_FB ==
  AI_MainHV_Minus_FB : Inport
  Constant : Constant  Value=IP_sFB_UB  OutDataTypeStr=single
  Constant1 : Constant  Value=IP_sFB_LB  OutDataTypeStr=single
  Constant2 : Constant  Value=IP_boActValue  OutDataTypeStr=boolean
  Constant3 : Constant  Value=IP_boDeactValue  OutDataTypeStr=boolean
  Constant4 : Constant  Value=IP_boInitValue  OutDataTypeStr=boolean
  Lib_Hysteresis_LowActive : Library_DataProcessing_v1_1/Lib_Hysteresis_LowActive  SystemSampleTime=-1  VariantActivationTime=update diagram  Latency=0  AutoFrameSizeCalculation=off
  IP_boHW_MainHV_Minus_FB : Outport
  wires:
  AI_MainHV_Minus_FB/1 -> Lib_Hysteresis_LowActive/1
  Lib_Hysteresis_LowActive/1 -> IP_boHW_MainHV_Minus_FB/1  "IP_boHW_MainHV_Minus_FB"
  Constant2/1 -> Lib_Hysteresis_LowActive/3
  Constant1/1 -> Lib_Hysteresis_LowActive/5
  Constant3/1 -> Lib_Hysteresis_LowActive/4
  Constant/1 -> Lib_Hysteresis_LowActive/6
  Constant4/1 -> Lib_Hysteresis_LowActive/2

== system ChiefMaster_TTC580/ChiefMaster/Input Processing/HW Inputs/Minuus_FB1 ==
  AI_DCHV_Minus_FB : Inport
  Constant : Constant  Value=IP_sFB_UB  OutDataTypeStr=single
  Constant1 : Constant  Value=IP_sFB_LB  OutDataTypeStr=single
  Constant2 : Constant  Value=IP_boActValue  OutDataTypeStr=boolean
  Constant3 : Constant  Value=IP_boDeactValue  OutDataTypeStr=boolean
  Constant4 : Constant  Value=IP_boInitValue  OutDataTypeStr=boolean
  Lib_Hysteresis_LowActive : Library_DataProcessing_v1_1/Lib_Hysteresis_LowActive  SystemSampleTime=-1  VariantActivationTime=update diagram  Latency=0  AutoFrameSizeCalculation=off
  IP_boHW_DCHV_Minus_FB : Outport
  wires:
  Lib_Hysteresis_LowActive/1 -> IP_boHW_DCHV_Minus_FB/1  "IP_boHW_DCHV_Minus_FB"
  AI_DCHV_Minus_FB/1 -> Lib_Hysteresis_LowActive/1
  Constant1/1 -> Lib_Hysteresis_LowActive/5
  Constant/1 -> Lib_Hysteresis_LowActive/6
  Constant3/1 -> Lib_Hysteresis_LowActive/4
  Constant2/1 -> Lib_Hysteresis_LowActive/3
  Constant4/1 -> Lib_Hysteresis_LowActive/2

== system ChiefMaster_TTC580/ChiefMaster/Input Processing/HW Inputs/Plus_FB ==
  AI_MainHV_Plus_FB : Inport
  Constant : Constant  Value=IP_sFB_UB  OutDataTypeStr=single
  Constant1 : Constant  Value=IP_sFB_LB  OutDataTypeStr=single
  Constant2 : Constant  Value=IP_boActValue  OutDataTypeStr=boolean
  Constant3 : Constant  Value=IP_boDeactValue  OutDataTypeStr=boolean
  Constant4 : Constant  Value=IP_boInitValue  OutDataTypeStr=boolean
  Lib_Hysteresis_LowActive : Library_DataProcessing_v1_1/Lib_Hysteresis_LowActive  SystemSampleTime=-1  VariantActivationTime=update diagram  Latency=0  AutoFrameSizeCalculation=off
  IP_boHW_MainHV_Plus_FB : Outport
  wires:
  Lib_Hysteresis_LowActive/1 -> IP_boHW_MainHV_Plus_FB/1  "IP_boHW_MainHV_Plus_FB"
  AI_MainHV_Plus_FB/1 -> Lib_Hysteresis_LowActive/1
  Constant/1 -> Lib_Hysteresis_LowActive/6
  Constant1/1 -> Lib_Hysteresis_LowActive/5
  Constant3/1 -> Lib_Hysteresis_LowActive/4
  Constant2/1 -> Lib_Hysteresis_LowActive/3
  Constant4/1 -> Lib_Hysteresis_LowActive/2

== system ChiefMaster_TTC580/ChiefMaster/Input Processing/HW Inputs/Plus_FB1 ==
  AI_DCHV_Plus_FB : Inport
  Constant : Constant  Value=IP_sFB_UB  OutDataTypeStr=single
  Constant1 : Constant  Value=IP_sFB_LB  OutDataTypeStr=single
  Constant2 : Constant  Value=IP_boActValue  OutDataTypeStr=boolean
  Constant3 : Constant  Value=IP_boDeactValue  OutDataTypeStr=boolean
  Constant4 : Constant  Value=IP_boInitValue  OutDataTypeStr=boolean
  Lib_Hysteresis_LowActive : Library_DataProcessing_v1_1/Lib_Hysteresis_LowActive  SystemSampleTime=-1  VariantActivationTime=update diagram  Latency=0  AutoFrameSizeCalculation=off
  IP_boHW_DCHV_Plus_FB : Outport
  wires:
  AI_DCHV_Plus_FB/1 -> Lib_Hysteresis_LowActive/1
  Lib_Hysteresis_LowActive/1 -> IP_boHW_DCHV_Plus_FB/1  "IP_boHW_DCHV_Plus_FB"
  Constant2/1 -> Lib_Hysteresis_LowActive/3
  Constant1/1 -> Lib_Hysteresis_LowActive/5
  Constant3/1 -> Lib_Hysteresis_LowActive/4
  Constant/1 -> Lib_Hysteresis_LowActive/6
  Constant4/1 -> Lib_Hysteresis_LowActive/2

== system ChiefMaster_TTC580/ChiefMaster/Input Processing/HW Inputs/Subsystem ==
  In : Inport
  Constant : Constant  Value=IP_u8HW_IN_delay_ms  OutDataTypeStr=uint16
  Input_Delay : Stateflow chart  TreatAsAtomicUnit=on
  Out : Outport
  wires:
  Constant/1 -> Input_Delay/1(IP_u8HW_IN_delay_ms)
  Input_Delay/1(out) -> Out/1
  In/1 -> Input_Delay/2(Input)

== system ChiefMaster_TTC580/ChiefMaster/Input Processing/HW Inputs/Subsystem1 ==
  DI_Proximity_BB2 : Inport
  Constant : Constant  Value=IP_u8HW_IN_delay_ms  OutDataTypeStr=uint16
  Input_Delay : Stateflow chart  TreatAsAtomicUnit=on
  Out : Outport
  wires:
  DI_Proximity_BB2/1 -> Input_Delay/2(Input)
  Input_Delay/1(out) -> Out/1
  Constant/1 -> Input_Delay/1(IP_u8HW_IN_delay_ms)

== system ChiefMaster_TTC580/ChiefMaster/Input Processing/HW Inputs/Subsystem2 ==
  DI_Proximity_BB2 : Inport
  Constant : Constant  Value=IP_u8HW_IN_delay_ms  OutDataTypeStr=uint16
  Input_Delay : Stateflow chart  TreatAsAtomicUnit=on
  Out : Outport
  wires:
  Constant/1 -> Input_Delay/1(IP_u8HW_IN_delay_ms)
  Input_Delay/1(out) -> Out/1
  DI_Proximity_BB2/1 -> Input_Delay/2(Input)

== system ChiefMaster_TTC580/ChiefMaster/Input Processing/LiBa/LiBa_Box1 ==
  C_LB_Batt1_CellVoltage01_Msg : Inport
  C_LB_Batt1_CellVoltage01_Timeout : Inport  Port=2
  C_LB_Batt1_CellVoltage02_Msg : Inport  Port=3
  C_LB_Batt1_CellVoltage02_Timeout : Inport  Port=4
  C_LB_Batt1_CellTemperature_Msg : Inport  Port=5
  C_LB_Batt1_CellTemperature_Timeout : Inport  Port=6
  C_LB_Batt1_InsulationMonitor_Msg : Inport  Port=7
  C_LB_Batt1_InsulationMonitor_Timeout : Inport  Port=8
  C_LB_Batt1_Status01_Msg : Inport  Port=9
  C_LB_Batt1_Status01_Timeout : Inport  Port=10
  C_LB_Batt1_Status02_Msg : Inport  Port=11
  C_LB_Batt1_Status02_Timeout : Inport  Port=12
  C_LB_Batt1_Status03_Msg : Inport  Port=13
  C_LB_Batt1_Status03_Timeout : Inport  Port=14
  BMS_CellTemperature : Subsystem
  BMS_CellVoltage01 : Subsystem
  BMS_CellVoltageNumber : Subsystem
  BMS_InsulationMonitor : Subsystem
  BMS_Status01 : Subsystem
  BMS_Status02 : Subsystem
  BMS_Status03 : Subsystem
  Bus Creator1 : BusCreator  Inputs=8
  Subsystem13 : Subsystem
  IP_LB_BattBox1_DataBus : Outport
  wires:
  C_LB_Batt1_CellVoltage01_Msg/1 -> BMS_CellVoltage01/1(C_LB_Batt1_CellVoltage01_Msg)
  C_LB_Batt1_CellVoltage01_Timeout/1 -> Subsystem13/1(C_LB_Batt1_CellVoltage01_Timeout), BMS_CellVoltage01/2(C_LB_Batt1_CellVoltage01_Timeout)
  C_LB_Batt1_CellVoltage02_Msg/1 -> BMS_CellVoltageNumber/1(C_LB_Batt1_CellVoltage02_Msg)
  C_LB_Batt1_CellVoltage02_Timeout/1 -> Subsystem13/2(C_LB_Batt1_CellVoltage02_Timeout), BMS_CellVoltageNumber/2(C_LB_Batt1_CellVoltage02_Timeout)
  BMS_CellVoltage01/1(IP_LB_Batt1_CellVoltage01_DataBus) -> Bus Creator1/1
  BMS_CellVoltageNumber/1(IP_LB_Batt1_CellVoltage02_DataBus) -> Bus Creator1/2
  Bus Creator1/1 -> IP_LB_BattBox1_DataBus/1  "IP_LB_BattBox1_DataBus"
  C_LB_Batt1_CellTemperature_Msg/1 -> BMS_CellTemperature/1(C_LB_Batt1_CellTemperature_Msg)
  C_LB_Batt1_CellTemperature_Timeout/1 -> BMS_CellTemperature/2(C_LB_Batt1_CellTemperature_Timeout), Subsystem13/3(C_LB_Batt1_CellTemperature_Timeout)
  BMS_CellTemperature/1(IP_LB_Batt1_CellTemperature_DataBus) -> Bus Creator1/3
  C_LB_Batt1_InsulationMonitor_Msg/1 -> BMS_InsulationMonitor/1(C_LB_Batt1_InsulationMonitor_Msg)
  C_LB_Batt1_InsulationMonitor_Timeout/1 -> BMS_InsulationMonitor/2(C_LB_Batt1_InsulationMonitor_Timeout), Subsystem13/4(C_LB_Batt1_InsulationMonitor_Timeout)
  BMS_InsulationMonitor/1(IP_LB_Batt1_InsulationMonitor_DataBus) -> Bus Creator1/4
  BMS_Status01/1(IP_LB_Batt1_Status01_DataBus) -> Bus Creator1/5
  C_LB_Batt1_Status01_Msg/1 -> BMS_Status01/1(C_LB_Batt1_Status01_Msg)
  C_LB_Batt1_Status01_Timeout/1 -> BMS_Status01/2(C_LB_Batt1_Status01_Timeout), Subsystem13/5(C_LB_Batt1_Status01_Timeout)
  C_LB_Batt1_Status02_Timeout/1 -> BMS_Status02/2(C_LB_Batt1_Status02_Timeout), Subsystem13/6(C_LB_Batt1_Status02_Timeout)
  C_LB_Batt1_Status02_Msg/1 -> BMS_Status02/1(C_LB_Batt1_Status02_Msg)
  BMS_Status02/1(IP_LB_Batt1_Status02_DataBus) -> Bus Creator1/6
  C_LB_Batt1_Status03_Msg/1 -> BMS_Status03/1(C_LB_Batt1_Status03_Msg)
  C_LB_Batt1_Status03_Timeout/1 -> BMS_Status03/2(C_LB_Batt1_Status03_Timeout), Subsystem13/7(C_LB_Batt1_Status03_Timeout)
  BMS_Status03/1(IP_LB_Batt1_Status03_DataBus) -> Bus Creator1/7
  Subsystem13/1(IP_boLiBa_Batt1_Availability) -> Bus Creator1/8

== system ChiefMaster_TTC580/ChiefMaster/Input Processing/LiBa/LiBa_Box2 ==
  C_LB_Batt2_CellVoltage01_Msg : Inport
  C_LB_Batt2_CellVoltage01_Timeout : Inport  Port=2
  C_LB_Batt2_CellVoltage02_Msg : Inport  Port=3
  C_LB_Batt2_CellVoltage02_Timeout : Inport  Port=4
  C_LB_Batt2_CellTemperature_Msg : Inport  Port=5
  C_LB_Batt2_CellTemperature_Timeout : Inport  Port=6
  C_LB_Batt2_InsulationMonitor_Msg : Inport  Port=7
  C_LB_Batt2_InsulationMonitor_Timeout : Inport  Port=8
  C_LB_Batt2_Status01_Msg : Inport  Port=9
  C_LB_Batt2_Status01_Timeout : Inport  Port=10
  C_LB_Batt2_Status02_Msg : Inport  Port=11
  C_LB_Batt2_Status02_Timeout : Inport  Port=12
  C_LB_Batt2_Status03_Msg : Inport  Port=13
  C_LB_Batt2_Status03_Timeout : Inport  Port=14
  BMS_CellTemperature : Subsystem
  BMS_CellVoltage01 : Subsystem
  BMS_CellVoltageNumber : Subsystem
  BMS_InsulationMonitor : Subsystem
  BMS_Status01 : Subsystem
  BMS_Status02 : Subsystem
  BMS_Status03 : Subsystem
  Bus Creator1 : BusCreator  Inputs=8
  Subsystem13 : Subsystem
  IP_LB_BattBox2_DataBus : Outport
  wires:
  C_LB_Batt2_CellVoltage01_Msg/1 -> BMS_CellVoltage01/1(C_LB_Batt2_CellVoltage01_Msg)
  C_LB_Batt2_CellVoltage01_Timeout/1 -> Subsystem13/1(C_LB_Batt1_CellVoltage01_Timeout), BMS_CellVoltage01/2(C_LB_Batt2_CellVoltage01_Timeout)
  C_LB_Batt2_CellVoltage02_Msg/1 -> BMS_CellVoltageNumber/1(C_LB_Batt2_CellVoltage02_Msg)
  C_LB_Batt2_CellVoltage02_Timeout/1 -> Subsystem13/2(C_LB_Batt1_CellVoltage02_Timeout), BMS_CellVoltageNumber/2(C_LB_Batt2_CellVoltage02_Timeout)
  BMS_CellVoltage01/1(IP_LB_Batt2_CellVoltage01_DataBus) -> Bus Creator1/1
  BMS_CellVoltageNumber/1(IP_LB_Batt2_CellVoltage02_DataBus) -> Bus Creator1/2
  Bus Creator1/1 -> IP_LB_BattBox2_DataBus/1  "IP_LB_BattBox2_DataBus"
  C_LB_Batt2_CellTemperature_Msg/1 -> BMS_CellTemperature/1(C_LB_Batt2_CellTemperature_Msg)
  C_LB_Batt2_CellTemperature_Timeout/1 -> Subsystem13/3(C_LB_Batt1_CellTemperature_Timeout), BMS_CellTemperature/2(C_LB_Batt2_CellTemperature_Timeout)
  BMS_CellTemperature/1(IP_LB_Batt2_CellTemperature_DataBus) -> Bus Creator1/3
  C_LB_Batt2_InsulationMonitor_Msg/1 -> BMS_InsulationMonitor/1(C_LB_Batt2_InsulationMonitor_Msg)
  C_LB_Batt2_InsulationMonitor_Timeout/1 -> BMS_InsulationMonitor/2(C_LB_Batt2_InsulationMonitor_Timeout), Subsystem13/4(C_LB_Batt1_InsulationMonitor_Timeout)
  BMS_InsulationMonitor/1(IP_LB_Batt2_InsulationMonitor_DataBus) -> Bus Creator1/4
  BMS_Status01/1(IP_LB_Batt2_Status01_DataBus) -> Bus Creator1/5
  C_LB_Batt2_Status01_Msg/1 -> BMS_Status01/1(C_LB_Batt2_Status01_Msg)
  C_LB_Batt2_Status01_Timeout/1 -> Subsystem13/5(C_LB_Batt1_Status01_Timeout), BMS_Status01/2(C_LB_Batt2_Status01_Timeout)
  C_LB_Batt2_Status02_Timeout/1 -> BMS_Status02/2(C_LB_Batt2_Status02_Timeout), Subsystem13/6(C_LB_Batt1_Status02_Timeout)
  C_LB_Batt2_Status02_Msg/1 -> BMS_Status02/1(C_LB_Batt2_Status02_Msg)
  BMS_Status02/1(IP_LB_Batt2_Status02_DataBus) -> Bus Creator1/6
  C_LB_Batt2_Status03_Msg/1 -> BMS_Status03/1(C_LB_Batt2_Status03_Msg)
  C_LB_Batt2_Status03_Timeout/1 -> BMS_Status03/2(C_LB_Batt2_Status03_Timeout), Subsystem13/7(C_LB_Batt1_Status03_Timeout)
  BMS_Status03/1(IP_LB_Batt2_Status03_DataBus) -> Bus Creator1/7
  Subsystem13/1(IP_boLiBa_Batt2_Availability) -> Bus Creator1/8

== system ChiefMaster_TTC580/ChiefMaster/Input Processing/LiBa/LiBa_Box3 ==
  C_LB_Batt3_CellVoltage01_Msg : Inport
  C_LB_Batt3_CellVoltage01_Timeout : Inport  Port=2
  C_LB_Batt3_CellVoltage02_Msg : Inport  Port=3
  C_LB_Batt3_CellVoltage02_Timeout : Inport  Port=4
  C_LB_Batt3_CellTemperature_Msg : Inport  Port=5
  C_LB_Batt3_CellTemperature_Timeout : Inport  Port=6
  C_LB_Batt3_InsulationMonitor_Msg : Inport  Port=7
  C_LB_Batt3_InsulationMonitor_Timeout : Inport  Port=8
  C_LB_Batt3_Status01_Msg : Inport  Port=9
  C_LB_Batt3_Status01_Timeout : Inport  Port=10
  C_LB_Batt3_Status02_Msg : Inport  Port=11
  C_LB_Batt3_Status02_Timeout : Inport  Port=12
  C_LB_Batt3_Status03_Msg : Inport  Port=13
  C_LB_Batt3_Status03_Timeout : Inport  Port=14
  BMS_CellTemperature : Subsystem
  BMS_CellVoltage01 : Subsystem
  BMS_CellVoltageNumber : Subsystem
  BMS_InsulationMonitor : Subsystem
  BMS_Status01 : Subsystem
  BMS_Status02 : Subsystem
  BMS_Status03 : Subsystem
  Bus Creator1 : BusCreator  Inputs=8
  Subsystem13 : Subsystem
  IP_LB_BattBox3_DataBus : Outport
  wires:
  C_LB_Batt3_CellVoltage01_Msg/1 -> BMS_CellVoltage01/1(C_LB_Batt3_CellVoltage01_Msg)
  C_LB_Batt3_CellVoltage01_Timeout/1 -> Subsystem13/1(C_LB_Batt1_CellVoltage01_Timeout), BMS_CellVoltage01/2(C_LB_Batt3_CellVoltage01_Timeout)
  C_LB_Batt3_CellVoltage02_Msg/1 -> BMS_CellVoltageNumber/1(C_LB_Batt3_CellVoltage02_Msg)
  C_LB_Batt3_CellVoltage02_Timeout/1 -> Subsystem13/2(C_LB_Batt1_CellVoltage02_Timeout), BMS_CellVoltageNumber/2(C_LB_Batt3_CellVoltage02_Timeout)
  BMS_CellVoltage01/1(IP_LB_Batt3_CellVoltage01_DataBus) -> Bus Creator1/1
  BMS_CellVoltageNumber/1(IP_LB_Batt3_CellVoltage02_DataBus) -> Bus Creator1/2
  Bus Creator1/1 -> IP_LB_BattBox3_DataBus/1  "IP_LB_BattBox3_DataBus"
  C_LB_Batt3_CellTemperature_Msg/1 -> BMS_CellTemperature/1(C_LB_Batt3_CellTemperature_Msg)
  C_LB_Batt3_CellTemperature_Timeout/1 -> Subsystem13/3(C_LB_Batt1_CellTemperature_Timeout), BMS_CellTemperature/2(C_LB_Batt3_CellTemperature_Timeout)
  BMS_CellTemperature/1(IP_LB_Batt3_CellTemperature_DataBus) -> Bus Creator1/3
  C_LB_Batt3_InsulationMonitor_Msg/1 -> BMS_InsulationMonitor/1(C_LB_Batt3_InsulationMonitor_Msg)
  C_LB_Batt3_InsulationMonitor_Timeout/1 -> Subsystem13/4(C_LB_Batt1_InsulationMonitor_Timeout), BMS_InsulationMonitor/2(C_LB_Batt3_InsulationMonitor_Timeout)
  BMS_InsulationMonitor/1(IP_LB_Batt3_InsulationMonitor_DataBus) -> Bus Creator1/4
  BMS_Status01/1(IP_LB_Batt3_Status01_DataBus) -> Bus Creator1/5
  C_LB_Batt3_Status01_Msg/1 -> BMS_Status01/1(C_LB_Batt3_Status01_Msg)
  C_LB_Batt3_Status01_Timeout/1 -> BMS_Status01/2(C_LB_Batt3_Status01_Timeout), Subsystem13/5(C_LB_Batt1_Status01_Timeout)
  C_LB_Batt3_Status02_Timeout/1 -> BMS_Status02/2(C_LB_Batt3_Status02_Timeout), Subsystem13/6(C_LB_Batt1_Status02_Timeout)
  C_LB_Batt3_Status02_Msg/1 -> BMS_Status02/1(C_LB_Batt3_Status02_Msg)
  BMS_Status02/1(IP_LB_Batt3_Status02_DataBus) -> Bus Creator1/6
  C_LB_Batt3_Status03_Msg/1 -> BMS_Status03/1(C_LB_Batt3_Status03_Msg)
  C_LB_Batt3_Status03_Timeout/1 -> BMS_Status03/2(C_LB_Batt3_Status03_Timeout), Subsystem13/7(C_LB_Batt1_Status03_Timeout)
  BMS_Status03/1("IP_LB_Batt3_Status03_DataBus ") -> Bus Creator1/7
  Subsystem13/1(IP_boLiBa_Batt3_Availability) -> Bus Creator1/8

== system ChiefMaster_TTC580/ChiefMaster/Input Processing/Subsystem2/Subsystem1 ==
  byte1 : Inport
  Timeout : EnablePort
  Bus Creator : BusCreator  Inputs=6
  Constant : Constant  OutDataTypeStr=boolean
  Data Type Conversion{2..8} (7 alike) : DataTypeConversion  OutDataTypeStr=boolean  SaturateOnIntegerOverflow=off  RndMeth=Floor
  Extract Bits : simulink/Logic and Bit Operations/Extract Bits  bitsToExtract=Range of bits  numBits=8  bitIdxRange=[0]  outScalingMode=Treat bit field as an integer
  Extract Bits1 : simulink/Logic and Bit Operations/Extract Bits  bitsToExtract=Range of bits  numBits=8  bitIdxRange=[1]  outScalingMode=Treat bit field as an integer
  Extract Bits2 : simulink/Logic and Bit Operations/Extract Bits  bitsToExtract=Range of bits  numBits=8  bitIdxRange=[2]  outScalingMode=Treat bit field as an integer
  Extract Bits3 : simulink/Logic and Bit Operations/Extract Bits  bitsToExtract=Range of bits  numBits=8  bitIdxRange=[3]  outScalingMode=Treat bit field as an integer
  Extract Bits4 : simulink/Logic and Bit Operations/Extract Bits  bitsToExtract=Range of bits  numBits=8  bitIdxRange=[4]  outScalingMode=Treat bit field as an integer
  Extract Bits5 : simulink/Logic and Bit Operations/Extract Bits  bitsToExtract=Range of bits  numBits=8  bitIdxRange=[5]  outScalingMode=Treat bit field as an integer
  Extract Bits6 : simulink/Logic and Bit Operations/Extract Bits  bitsToExtract=Range of bits  numBits=8  bitIdxRange=[6]  outScalingMode=Treat bit field as an integer
  Terminator1 : Terminator
  Terminator5 : Terminator
  TTC_Status_Databus : Outport  OutputWhenDisabled=reset  InitialOutput=[0]
  wires:
  Extract Bits5/1 -> Data Type Conversion7/1
  byte1/1 -> Extract Bits4/1, Extract Bits5/1, Extract Bits6/1, Extract Bits/1, Extract Bits1/1, Extract Bits2/1, Extract Bits3/1
  Extract Bits3/1 -> Data Type Conversion5/1
  Extract Bits6/1 -> Data Type Conversion8/1
  Extract Bits/1 -> Data Type Conversion2/1
  Extract Bits1/1 -> Data Type Conversion3/1
  Extract Bits4/1 -> Data Type Conversion6/1
  Extract Bits2/1 -> Data Type Conversion4/1
  Data Type Conversion2/1 -> Bus Creator/1  "IP_boSafeToShutdown"
  Bus Creator/1 -> TTC_Status_Databus/1  "TTC_Status_Databus"
  Data Type Conversion3/1 -> Bus Creator/2  "IP_boKL15_D"
  Data Type Conversion4/1 -> Bus Creator/3  "IP_boKL15_C"
  Data Type Conversion5/1 -> Bus Creator/4  "IP_boEVDisconnectingDevice"
  Constant/1 -> Bus Creator/5  "IP_boEV_IsolationMeasurementRequest"
  Data Type Conversion7/1 -> Bus Creator/6  "IP_boChargeStop_Button"
  Data Type Conversion8/1 -> Terminator5/1
  Data Type Conversion6/1 -> Terminator1/1  "IP_boEV_IsolationMeasurementRequest"

== system ChiefMaster_TTC580/ChiefMaster/Input Processing/Subsystem2/Subsystem3 ==
  byte2 : Inport
  byte3 : Inport  Port=2
  C_TTC_Msg1_Timeout : Inport  Port=3
  Bus Creator : BusCreator  Inputs=3
  Constant : Constant  Value=IP_sLoad_Voltage_Factor  OutDataTypeStr=single
  Constant1 : Constant  Value=IP_sLoad_Voltage_Offset  OutDataTypeStr=single
  Constant2 : Constant  Value=IP_sLoad_Voltage_LB  OutDataTypeStr=single
  Constant3 : Constant  Value=IP_sLoad_Voltage_UB  OutDataTypeStr=single
  Lib_2byte_ArthConcat : Library_DataProcessing_v1/Lib_2byte_ArthConcat  SystemSampleTime=-1  VariantActivationTime=update diagram  Latency=0  AutoFrameSizeCalculation=off
  Lib_InputProcessing+SafeValueSelector_Data : Library_DataProcessing_v1/Lib_InputProcessing+SafeValueSelector_Data  SystemSampleTime=-1  VariantActivationTime=update diagram  Latency=0  AutoFrameSizeCalculation=off
  SafeValue_Error : Constant  Priority=1005  Value=0  OutDataTypeStr=single
  "SafeValue_NA " : Constant  Priority=1006  Value=0  OutDataTypeStr=single
  IP_sLoadVoltage_Databus : Outport
  wires:
  Bus Creator/1 -> IP_sLoadVoltage_Databus/1  "IP_sLoadVoltage_Databus"
  byte2/1 -> Lib_2byte_ArthConcat/1
  byte3/1 -> Lib_2byte_ArthConcat/2
  Constant1/1 -> Lib_InputProcessing+SafeValueSelector_Data/4
  Constant/1 -> Lib_InputProcessing+SafeValueSelector_Data/3
  Constant2/1 -> Lib_InputProcessing+SafeValueSelector_Data/5
  Constant3/1 -> Lib_InputProcessing+SafeValueSelector_Data/6
  Lib_InputProcessing+SafeValueSelector_Data/3 -> Bus Creator/3
  Lib_InputProcessing+SafeValueSelector_Data/2 -> Bus Creator/2
  SafeValue_Error/1 -> Lib_InputProcessing+SafeValueSelector_Data/7
  Lib_InputProcessing+SafeValueSelector_Data/1 -> Bus Creator/1
  "SafeValue_NA "/1 -> Lib_InputProcessing+SafeValueSelector_Data/8
  C_TTC_Msg1_Timeout/1 -> Lib_InputProcessing+SafeValueSelector_Data/2
  Lib_2byte_ArthConcat/1 -> Lib_InputProcessing+SafeValueSelector_Data/1
